simulink model "Pianta"  (R2025b)
settings: Solver=VariableStepAuto  StartTime=0.0  StopTime=100.0  RelTol=1e-3
values from neighbouring files (symbols this model uses):
  Gb = 119.1858    [fase1.m]
  Ib = 15.3872    [fase1.m]
  p1 = 0.0287    [fase1.m]
  p2 = 0.0283    [fase1.m]
  p3 = 5.035*10^(-5)    (= 5.035e-05)    [fase1.m]
  p4 = 5/54    (= 0.0925925925926)    [fase1.m]
settings Model: Creator=Rika  LastModifiedBy=Rika
settings DataIOCC: ExternalInput=[0 0 0]  InitialState=[]  LoadExternalInput=on  LoadInitialState=on
settings OptimizationCC: DefaultParameterBehavior=Inlined  BufferReuse=off
settings DebuggingCC: InitInArrayFormatMsg=none

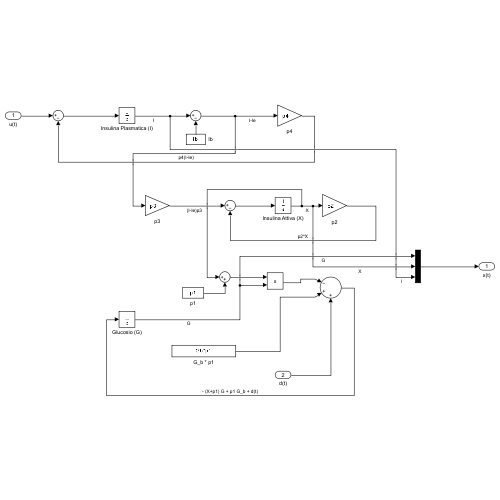
[thumbnail: Simulink's stored preview of the top-level diagram]
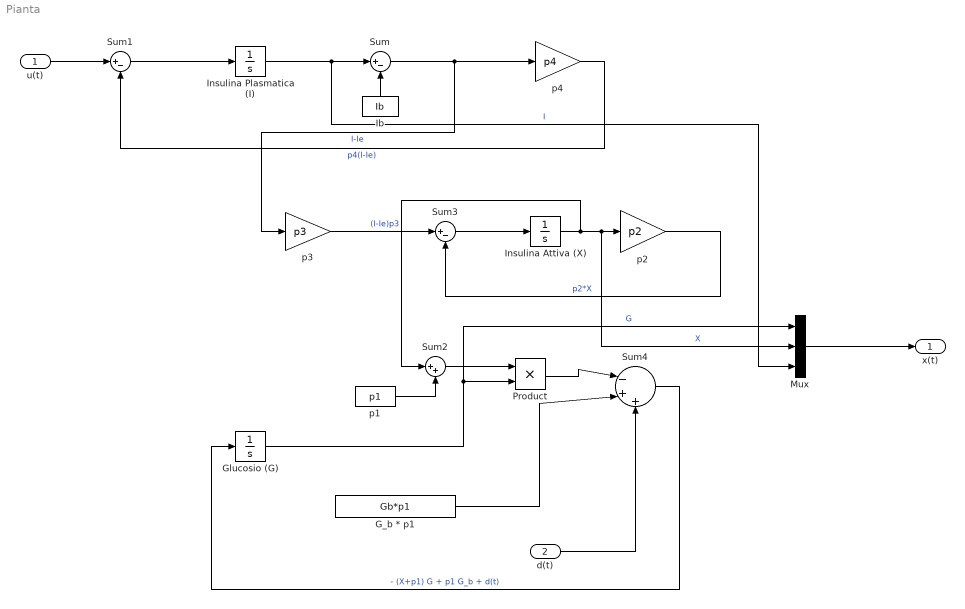
== system Pianta ==
  u(t) : Inport
  d(t) : Inport  Port=2
  G_b * p1 : Constant  Value=Gb*p1
  Glucosio (G) : Integrator  InitialCondition=119.1858
  Ib : Constant  Value=Ib
  Insulina Attiva (X) : Integrator
  Insulina Plasmatica (I) : Integrator  InitialCondition=15.3872
  Mux : Mux  Inputs=3
  Product : Product
  Sum : Sum  Inputs=|+-
  Sum1 : Sum  Inputs=|+-
  Sum2 : Sum  Inputs=|++
  Sum3 : Sum  Inputs=|+-
  Sum4 : Sum  Inputs=|-++
  p1 : Constant  Value=p1
  p2 : Gain  Gain=p2
  p3 : Gain  Gain=p3
  p4 : Gain  Gain=p4
  x(t) : Outport
  wires:
  Ib/1 -> Sum/2
  Insulina Plasmatica (I)/1 -> Mux/3, Sum/1  "I"
  Sum/1 -> p4/1, p3/1  "I-Ie"
  Sum1/1 -> Insulina Plasmatica (I)/1
  p4/1 -> Sum1/2  "p4(I-Ie)"
  Insulina Attiva (X)/1 -> Sum2/1, Mux/2, p2/1  "X"
  p3/1 -> Sum3/1  "(I-Ie)p3"
  p2/1 -> Sum3/2  "p2*X"
  Sum3/1 -> Insulina Attiva (X)/1
  p1/1 -> Sum2/2
  Sum2/1 -> Product/1
  Glucosio (G)/1 -> Mux/1, Product/2  "G"
  G_b * p1/1 -> Sum4/2
  Sum4/1 -> Glucosio (G)/1  "- (X+p1) G + p1 G_b + d(t)"
  u(t)/1 -> Sum1/1
  Product/1 -> Sum4/1
  d(t)/1 -> Sum4/3
  Mux/1 -> x(t)/1
